simulink model "Aloe_E_Cell_Project"  (R2019b)
settings: Solver=VariableStepAuto  StartTime=0.0  StopTime=0.14  RelTol=1e-3
undefined symbols (not defined in the file): D1, Delta
libraries: powerlib x218, powerlib_meascontrol x6, simulink x2
(part 2 of 3)

== system Aloe_E_Cell_Project/Aloe E Battery Array/12 V Aloe E-Cell23 ==
  Constant : Constant  Value=4
  Constant1 : Constant  Value=24
  Controlled Current Source : powerlib/Electrical Sources/Controlled Current Source  Initialize=on  Source_Type=DC  Amplitude=1  Phase=0  Frequency=0  Measurements=None
      settings: SourceProductName=Simscape Electrical
  Controlled Voltage Source : powerlib/Electrical Sources/Controlled Voltage Source  Initialize=on  Source_Type=DC  Amplitude=1  Phase=0  Frequency=0  Measurements=Voltage
      settings: SourceProductName=Simscape Electrical
  Current Measurement : powerlib/Measurements/Current Measurement  PhasorSimulation=off  OutputType=Complex  PSBequivalent=0
      settings: SourceProductName=Simscape Electrical
  Display : Display
      settings: Decimation=3
  Display1 : Display
      settings: Decimation=3
  Series RLC Branch1 : powerlib/Elements/Series RLC Branch  LConnTagsString=__new0  RConnTagsString=__new0  BranchType=R  Resistance=6  Inductance=1e-3  SetiL0=off  InitialCurrent=0  Capacitance=1e-6  Setx0=off  InitialVoltage=0  Measurements=None
      settings: SourceProductName=Simscape Electrical
  Voltage Measurement : powerlib/Measurements/Voltage Measurement  PhasorSimulation=off  OutputType=Complex  PSBequivalent=0
      settings: SourceProductName=Simscape Electrical
  V+ : PMIOPort  Side=Right
  "V- " : PMIOPort  Port=2  Side=Right
  wires:
  Constant/1 -> Controlled Current Source/1
  Constant1/1 -> Controlled Voltage Source/1
  Current Measurement/1 -> Display1/1
  Voltage Measurement/1 -> Display/1
  connections:
  Series RLC Branch1/LConn1 -- Current Measurement/RConn1 -- Voltage Measurement/LConn1 -- V+/RConn1
  Controlled Voltage Source/RConn1 -- Controlled Current Source/LConn1
  Controlled Voltage Source/LConn1 -- Series RLC Branch1/RConn1 -- Voltage Measurement/LConn2 -- "V- "/RConn1
  Controlled Current Source/RConn1 -- Current Measurement/LConn1

== system Aloe_E_Cell_Project/Aloe E Battery Array/12 V Aloe E-Cell24 ==
  Constant : Constant  Value=4
  Constant1 : Constant  Value=24
  Controlled Current Source : powerlib/Electrical Sources/Controlled Current Source  Initialize=on  Source_Type=DC  Amplitude=1  Phase=0  Frequency=0  Measurements=None
      settings: SourceProductName=Simscape Electrical
  Controlled Voltage Source : powerlib/Electrical Sources/Controlled Voltage Source  Initialize=on  Source_Type=DC  Amplitude=1  Phase=0  Frequency=0  Measurements=Voltage
      settings: SourceProductName=Simscape Electrical
  Current Measurement : powerlib/Measurements/Current Measurement  PhasorSimulation=off  OutputType=Complex  PSBequivalent=0
      settings: SourceProductName=Simscape Electrical
  Display : Display
      settings: Decimation=3
  Display1 : Display
      settings: Decimation=3
  Series RLC Branch1 : powerlib/Elements/Series RLC Branch  LConnTagsString=__new0  RConnTagsString=__new0  BranchType=R  Resistance=6  Inductance=1e-3  SetiL0=off  InitialCurrent=0  Capacitance=1e-6  Setx0=off  InitialVoltage=0  Measurements=None
      settings: SourceProductName=Simscape Electrical
  Voltage Measurement : powerlib/Measurements/Voltage Measurement  PhasorSimulation=off  OutputType=Complex  PSBequivalent=0
      settings: SourceProductName=Simscape Electrical
  V+ : PMIOPort  Side=Right
  "V- " : PMIOPort  Port=2  Side=Right
  wires:
  Voltage Measurement/1 -> Display/1
  Current Measurement/1 -> Display1/1
  Constant1/1 -> Controlled Voltage Source/1
  Constant/1 -> Controlled Current Source/1
  connections:
  Controlled Current Source/RConn1 -- Current Measurement/LConn1
  "V- "/RConn1 -- Voltage Measurement/LConn2 -- Series RLC Branch1/RConn1 -- Controlled Voltage Source/LConn1
  Controlled Voltage Source/RConn1 -- Controlled Current Source/LConn1
  V+/RConn1 -- Voltage Measurement/LConn1 -- Current Measurement/RConn1 -- Series RLC Branch1/LConn1

== system Aloe_E_Cell_Project/Aloe E Battery Array/12 V Aloe E-Cell25 ==
  Constant : Constant  Value=4
  Constant1 : Constant  Value=24
  Controlled Current Source : powerlib/Electrical Sources/Controlled Current Source  Initialize=on  Source_Type=DC  Amplitude=1  Phase=0  Frequency=0  Measurements=None
      settings: SourceProductName=Simscape Electrical
  Controlled Voltage Source : powerlib/Electrical Sources/Controlled Voltage Source  Initialize=on  Source_Type=DC  Amplitude=1  Phase=0  Frequency=0  Measurements=Voltage
      settings: SourceProductName=Simscape Electrical
  Current Measurement : powerlib/Measurements/Current Measurement  PhasorSimulation=off  OutputType=Complex  PSBequivalent=0
      settings: SourceProductName=Simscape Electrical
  Display : Display
      settings: Decimation=3
  Display1 : Display
      settings: Decimation=3
  Series RLC Branch1 : powerlib/Elements/Series RLC Branch  LConnTagsString=__new0  RConnTagsString=__new0  BranchType=R  Resistance=6  Inductance=1e-3  SetiL0=off  InitialCurrent=0  Capacitance=1e-6  Setx0=off  InitialVoltage=0  Measurements=None
      settings: SourceProductName=Simscape Electrical
  Voltage Measurement : powerlib/Measurements/Voltage Measurement  PhasorSimulation=off  OutputType=Complex  PSBequivalent=0
      settings: SourceProductName=Simscape Electrical
  V+ : PMIOPort  Side=Right
  "V- " : PMIOPort  Port=2  Side=Right
  wires:
  Voltage Measurement/1 -> Display/1
  Current Measurement/1 -> Display1/1
  Constant1/1 -> Controlled Voltage Source/1
  Constant/1 -> Controlled Current Source/1
  connections:
  Controlled Current Source/RConn1 -- Current Measurement/LConn1
  "V- "/RConn1 -- Voltage Measurement/LConn2 -- Series RLC Branch1/RConn1 -- Controlled Voltage Source/LConn1
  Controlled Voltage Source/RConn1 -- Controlled Current Source/LConn1
  V+/RConn1 -- Voltage Measurement/LConn1 -- Current Measurement/RConn1 -- Series RLC Branch1/LConn1

== system Aloe_E_Cell_Project/Aloe E Battery Array/12 V Aloe E-Cell26 ==
  Constant : Constant  Value=4
  Constant1 : Constant  Value=24
  Controlled Current Source : powerlib/Electrical Sources/Controlled Current Source  Initialize=on  Source_Type=DC  Amplitude=1  Phase=0  Frequency=0  Measurements=None
      settings: SourceProductName=Simscape Electrical
  Controlled Voltage Source : powerlib/Electrical Sources/Controlled Voltage Source  Initialize=on  Source_Type=DC  Amplitude=1  Phase=0  Frequency=0  Measurements=Voltage
      settings: SourceProductName=Simscape Electrical
  Current Measurement : powerlib/Measurements/Current Measurement  PhasorSimulation=off  OutputType=Complex  PSBequivalent=0
      settings: SourceProductName=Simscape Electrical
  Display : Display
      settings: Decimation=3
  Display1 : Display
      settings: Decimation=3
  Series RLC Branch1 : powerlib/Elements/Series RLC Branch  LConnTagsString=__new0  RConnTagsString=__new0  BranchType=R  Resistance=6  Inductance=1e-3  SetiL0=off  InitialCurrent=0  Capacitance=1e-6  Setx0=off  InitialVoltage=0  Measurements=None
      settings: SourceProductName=Simscape Electrical
  Voltage Measurement : powerlib/Measurements/Voltage Measurement  PhasorSimulation=off  OutputType=Complex  PSBequivalent=0
      settings: SourceProductName=Simscape Electrical
  V+ : PMIOPort  Side=Right
  "V- " : PMIOPort  Port=2  Side=Right
  wires:
  Constant/1 -> Controlled Current Source/1
  Constant1/1 -> Controlled Voltage Source/1
  Current Measurement/1 -> Display1/1
  Voltage Measurement/1 -> Display/1
  connections:
  Series RLC Branch1/LConn1 -- Current Measurement/RConn1 -- Voltage Measurement/LConn1 -- V+/RConn1
  Controlled Voltage Source/RConn1 -- Controlled Current Source/LConn1
  Controlled Voltage Source/LConn1 -- Series RLC Branch1/RConn1 -- Voltage Measurement/LConn2 -- "V- "/RConn1
  Controlled Current Source/RConn1 -- Current Measurement/LConn1

== system Aloe_E_Cell_Project/Aloe E Battery Array/12 V Aloe E-Cell27 ==
  Constant : Constant  Value=4
  Constant1 : Constant  Value=24
  Controlled Current Source : powerlib/Electrical Sources/Controlled Current Source  Initialize=on  Source_Type=DC  Amplitude=1  Phase=0  Frequency=0  Measurements=None
      settings: SourceProductName=Simscape Electrical
  Controlled Voltage Source : powerlib/Electrical Sources/Controlled Voltage Source  Initialize=on  Source_Type=DC  Amplitude=1  Phase=0  Frequency=0  Measurements=Voltage
      settings: SourceProductName=Simscape Electrical
  Current Measurement : powerlib/Measurements/Current Measurement  PhasorSimulation=off  OutputType=Complex  PSBequivalent=0
      settings: SourceProductName=Simscape Electrical
  Display : Display
      settings: Decimation=3
  Display1 : Display
      settings: Decimation=3
  Series RLC Branch1 : powerlib/Elements/Series RLC Branch  LConnTagsString=__new0  RConnTagsString=__new0  BranchType=R  Resistance=6  Inductance=1e-3  SetiL0=off  InitialCurrent=0  Capacitance=1e-6  Setx0=off  InitialVoltage=0  Measurements=None
      settings: SourceProductName=Simscape Electrical
  Voltage Measurement : powerlib/Measurements/Voltage Measurement  PhasorSimulation=off  OutputType=Complex  PSBequivalent=0
      settings: SourceProductName=Simscape Electrical
  V+ : PMIOPort  Side=Right
  "V- " : PMIOPort  Port=2  Side=Right
  wires:
  Voltage Measurement/1 -> Display/1
  Current Measurement/1 -> Display1/1
  Constant1/1 -> Controlled Voltage Source/1
  Constant/1 -> Controlled Current Source/1
  connections:
  Controlled Current Source/RConn1 -- Current Measurement/LConn1
  "V- "/RConn1 -- Voltage Measurement/LConn2 -- Series RLC Branch1/RConn1 -- Controlled Voltage Source/LConn1
  Controlled Voltage Source/RConn1 -- Controlled Current Source/LConn1
  V+/RConn1 -- Voltage Measurement/LConn1 -- Current Measurement/RConn1 -- Series RLC Branch1/LConn1

== system Aloe_E_Cell_Project/Aloe E Battery Array/12 V Aloe E-Cell28 ==
  Constant : Constant  Value=4
  Constant1 : Constant  Value=24
  Controlled Current Source : powerlib/Electrical Sources/Controlled Current Source  Initialize=on  Source_Type=DC  Amplitude=1  Phase=0  Frequency=0  Measurements=None
      settings: SourceProductName=Simscape Electrical
  Controlled Voltage Source : powerlib/Electrical Sources/Controlled Voltage Source  Initialize=on  Source_Type=DC  Amplitude=1  Phase=0  Frequency=0  Measurements=Voltage
      settings: SourceProductName=Simscape Electrical
  Current Measurement : powerlib/Measurements/Current Measurement  PhasorSimulation=off  OutputType=Complex  PSBequivalent=0
      settings: SourceProductName=Simscape Electrical
  Display : Display
      settings: Decimation=3
  Display1 : Display
      settings: Decimation=3
  Series RLC Branch1 : powerlib/Elements/Series RLC Branch  LConnTagsString=__new0  RConnTagsString=__new0  BranchType=R  Resistance=6  Inductance=1e-3  SetiL0=off  InitialCurrent=0  Capacitance=1e-6  Setx0=off  InitialVoltage=0  Measurements=None
      settings: SourceProductName=Simscape Electrical
  Voltage Measurement : powerlib/Measurements/Voltage Measurement  PhasorSimulation=off  OutputType=Complex  PSBequivalent=0
      settings: SourceProductName=Simscape Electrical
  V+ : PMIOPort  Side=Right
  "V- " : PMIOPort  Port=2  Side=Right
  wires:
  Voltage Measurement/1 -> Display/1
  Current Measurement/1 -> Display1/1
  Constant1/1 -> Controlled Voltage Source/1
  Constant/1 -> Controlled Current Source/1
  connections:
  Controlled Current Source/RConn1 -- Current Measurement/LConn1
  "V- "/RConn1 -- Voltage Measurement/LConn2 -- Series RLC Branch1/RConn1 -- Controlled Voltage Source/LConn1
  Controlled Voltage Source/RConn1 -- Controlled Current Source/LConn1
  V+/RConn1 -- Voltage Measurement/LConn1 -- Current Measurement/RConn1 -- Series RLC Branch1/LConn1

== system Aloe_E_Cell_Project/Aloe E Battery Array/12 V Aloe E-Cell29 ==
  Constant : Constant  Value=4
  Constant1 : Constant  Value=24
  Controlled Current Source : powerlib/Electrical Sources/Controlled Current Source  Initialize=on  Source_Type=DC  Amplitude=1  Phase=0  Frequency=0  Measurements=None
      settings: SourceProductName=Simscape Electrical
  Controlled Voltage Source : powerlib/Electrical Sources/Controlled Voltage Source  Initialize=on  Source_Type=DC  Amplitude=1  Phase=0  Frequency=0  Measurements=Voltage
      settings: SourceProductName=Simscape Electrical
  Current Measurement : powerlib/Measurements/Current Measurement  PhasorSimulation=off  OutputType=Complex  PSBequivalent=0
      settings: SourceProductName=Simscape Electrical
  Display : Display
      settings: Decimation=3
  Display1 : Display
      settings: Decimation=3
  Series RLC Branch1 : powerlib/Elements/Series RLC Branch  LConnTagsString=__new0  RConnTagsString=__new0  BranchType=R  Resistance=6  Inductance=1e-3  SetiL0=off  InitialCurrent=0  Capacitance=1e-6  Setx0=off  InitialVoltage=0  Measurements=None
      settings: SourceProductName=Simscape Electrical
  Voltage Measurement : powerlib/Measurements/Voltage Measurement  PhasorSimulation=off  OutputType=Complex  PSBequivalent=0
      settings: SourceProductName=Simscape Electrical
  V+ : PMIOPort  Side=Right
  "V- " : PMIOPort  Port=2  Side=Right
  wires:
  Constant/1 -> Controlled Current Source/1
  Constant1/1 -> Controlled Voltage Source/1
  Current Measurement/1 -> Display1/1
  Voltage Measurement/1 -> Display/1
  connections:
  Series RLC Branch1/LConn1 -- Current Measurement/RConn1 -- Voltage Measurement/LConn1 -- V+/RConn1
  Controlled Voltage Source/RConn1 -- Controlled Current Source/LConn1
  Controlled Voltage Source/LConn1 -- Series RLC Branch1/RConn1 -- Voltage Measurement/LConn2 -- "V- "/RConn1
  Controlled Current Source/RConn1 -- Current Measurement/LConn1

== system Aloe_E_Cell_Project/Aloe E Battery Array/12 V Aloe E-Cell3 ==
  Constant : Constant  Value=4
  Constant1 : Constant  Value=24
  Controlled Current Source : powerlib/Electrical Sources/Controlled Current Source  Initialize=on  Source_Type=DC  Amplitude=1  Phase=0  Frequency=0  Measurements=None
      settings: SourceProductName=Simscape Electrical
  Controlled Voltage Source : powerlib/Electrical Sources/Controlled Voltage Source  Initialize=on  Source_Type=DC  Amplitude=1  Phase=0  Frequency=0  Measurements=Voltage
      settings: SourceProductName=Simscape Electrical
  Current Measurement : powerlib/Measurements/Current Measurement  PhasorSimulation=off  OutputType=Complex  PSBequivalent=0
      settings: SourceProductName=Simscape Electrical
  Display : Display
      settings: Decimation=3
  Display1 : Display
      settings: Decimation=3
  Series RLC Branch1 : powerlib/Elements/Series RLC Branch  LConnTagsString=__new0  RConnTagsString=__new0  BranchType=R  Resistance=6  Inductance=1e-3  SetiL0=off  InitialCurrent=0  Capacitance=1e-6  Setx0=off  InitialVoltage=0  Measurements=None
      settings: SourceProductName=Simscape Electrical
  Voltage Measurement : powerlib/Measurements/Voltage Measurement  PhasorSimulation=off  OutputType=Complex  PSBequivalent=0
      settings: SourceProductName=Simscape Electrical
  V+ : PMIOPort  Side=Right
  "V- " : PMIOPort  Port=2  Side=Right
  wires:
  Constant/1 -> Controlled Current Source/1
  Constant1/1 -> Controlled Voltage Source/1
  Current Measurement/1 -> Display1/1
  Voltage Measurement/1 -> Display/1
  connections:
  Series RLC Branch1/LConn1 -- Current Measurement/RConn1 -- Voltage Measurement/LConn1 -- V+/RConn1
  Controlled Voltage Source/RConn1 -- Controlled Current Source/LConn1
  Controlled Voltage Source/LConn1 -- Series RLC Branch1/RConn1 -- Voltage Measurement/LConn2 -- "V- "/RConn1
  Controlled Current Source/RConn1 -- Current Measurement/LConn1

== system Aloe_E_Cell_Project/Aloe E Battery Array/12 V Aloe E-Cell30 ==
  Constant : Constant  Value=4
  Constant1 : Constant  Value=24
  Controlled Current Source : powerlib/Electrical Sources/Controlled Current Source  Initialize=on  Source_Type=DC  Amplitude=1  Phase=0  Frequency=0  Measurements=None
      settings: SourceProductName=Simscape Electrical
  Controlled Voltage Source : powerlib/Electrical Sources/Controlled Voltage Source  Initialize=on  Source_Type=DC  Amplitude=1  Phase=0  Frequency=0  Measurements=Voltage
      settings: SourceProductName=Simscape Electrical
  Current Measurement : powerlib/Measurements/Current Measurement  PhasorSimulation=off  OutputType=Complex  PSBequivalent=0
      settings: SourceProductName=Simscape Electrical
  Display : Display
      settings: Decimation=3
  Display1 : Display
      settings: Decimation=3
  Series RLC Branch1 : powerlib/Elements/Series RLC Branch  LConnTagsString=__new0  RConnTagsString=__new0  BranchType=R  Resistance=6  Inductance=1e-3  SetiL0=off  InitialCurrent=0  Capacitance=1e-6  Setx0=off  InitialVoltage=0  Measurements=None
      settings: SourceProductName=Simscape Electrical
  Voltage Measurement : powerlib/Measurements/Voltage Measurement  PhasorSimulation=off  OutputType=Complex  PSBequivalent=0
      settings: SourceProductName=Simscape Electrical
  V+ : PMIOPort  Side=Right
  "V- " : PMIOPort  Port=2  Side=Right
  wires:
  Constant/1 -> Controlled Current Source/1
  Constant1/1 -> Controlled Voltage Source/1
  Current Measurement/1 -> Display1/1
  Voltage Measurement/1 -> Display/1
  connections:
  Series RLC Branch1/LConn1 -- Current Measurement/RConn1 -- Voltage Measurement/LConn1 -- V+/RConn1
  Controlled Voltage Source/RConn1 -- Controlled Current Source/LConn1
  Controlled Voltage Source/LConn1 -- Series RLC Branch1/RConn1 -- Voltage Measurement/LConn2 -- "V- "/RConn1
  Controlled Current Source/RConn1 -- Current Measurement/LConn1

== system Aloe_E_Cell_Project/Aloe E Battery Array/12 V Aloe E-Cell31 ==
  Constant : Constant  Value=4
  Constant1 : Constant  Value=24
  Controlled Current Source : powerlib/Electrical Sources/Controlled Current Source  Initialize=on  Source_Type=DC  Amplitude=1  Phase=0  Frequency=0  Measurements=None
      settings: SourceProductName=Simscape Electrical
  Controlled Voltage Source : powerlib/Electrical Sources/Controlled Voltage Source  Initialize=on  Source_Type=DC  Amplitude=1  Phase=0  Frequency=0  Measurements=Voltage
      settings: SourceProductName=Simscape Electrical
  Current Measurement : powerlib/Measurements/Current Measurement  PhasorSimulation=off  OutputType=Complex  PSBequivalent=0
      settings: SourceProductName=Simscape Electrical
  Display : Display
      settings: Decimation=3
  Display1 : Display
      settings: Decimation=3
  Series RLC Branch1 : powerlib/Elements/Series RLC Branch  LConnTagsString=__new0  RConnTagsString=__new0  BranchType=R  Resistance=6  Inductance=1e-3  SetiL0=off  InitialCurrent=0  Capacitance=1e-6  Setx0=off  InitialVoltage=0  Measurements=None
      settings: SourceProductName=Simscape Electrical
  Voltage Measurement : powerlib/Measurements/Voltage Measurement  PhasorSimulation=off  OutputType=Complex  PSBequivalent=0
      settings: SourceProductName=Simscape Electrical
  V+ : PMIOPort  Side=Right
  "V- " : PMIOPort  Port=2  Side=Right
  wires:
  Voltage Measurement/1 -> Display/1
  Current Measurement/1 -> Display1/1
  Constant1/1 -> Controlled Voltage Source/1
  Constant/1 -> Controlled Current Source/1
  connections:
  Controlled Current Source/RConn1 -- Current Measurement/LConn1
  "V- "/RConn1 -- Voltage Measurement/LConn2 -- Series RLC Branch1/RConn1 -- Controlled Voltage Source/LConn1
  Controlled Voltage Source/RConn1 -- Controlled Current Source/LConn1
  V+/RConn1 -- Voltage Measurement/LConn1 -- Current Measurement/RConn1 -- Series RLC Branch1/LConn1

== system Aloe_E_Cell_Project/Aloe E Battery Array/12 V Aloe E-Cell32 ==
  Constant : Constant  Value=4
  Constant1 : Constant  Value=24
  Controlled Current Source : powerlib/Electrical Sources/Controlled Current Source  Initialize=on  Source_Type=DC  Amplitude=1  Phase=0  Frequency=0  Measurements=None
      settings: SourceProductName=Simscape Electrical
  Controlled Voltage Source : powerlib/Electrical Sources/Controlled Voltage Source  Initialize=on  Source_Type=DC  Amplitude=1  Phase=0  Frequency=0  Measurements=Voltage
      settings: SourceProductName=Simscape Electrical
  Current Measurement : powerlib/Measurements/Current Measurement  PhasorSimulation=off  OutputType=Complex  PSBequivalent=0
      settings: SourceProductName=Simscape Electrical
  Display : Display
      settings: Decimation=3
  Display1 : Display
      settings: Decimation=3
  Series RLC Branch1 : powerlib/Elements/Series RLC Branch  LConnTagsString=__new0  RConnTagsString=__new0  BranchType=R  Resistance=6  Inductance=1e-3  SetiL0=off  InitialCurrent=0  Capacitance=1e-6  Setx0=off  InitialVoltage=0  Measurements=None
      settings: SourceProductName=Simscape Electrical
  Voltage Measurement : powerlib/Measurements/Voltage Measurement  PhasorSimulation=off  OutputType=Complex  PSBequivalent=0
      settings: SourceProductName=Simscape Electrical
  V+ : PMIOPort  Side=Right
  "V- " : PMIOPort  Port=2  Side=Right
  wires:
  Constant/1 -> Controlled Current Source/1
  Constant1/1 -> Controlled Voltage Source/1
  Current Measurement/1 -> Display1/1
  Voltage Measurement/1 -> Display/1
  connections:
  Series RLC Branch1/LConn1 -- Current Measurement/RConn1 -- Voltage Measurement/LConn1 -- V+/RConn1
  Controlled Voltage Source/RConn1 -- Controlled Current Source/LConn1
  Controlled Voltage Source/LConn1 -- Series RLC Branch1/RConn1 -- Voltage Measurement/LConn2 -- "V- "/RConn1
  Controlled Current Source/RConn1 -- Current Measurement/LConn1

== system Aloe_E_Cell_Project/Aloe E Battery Array/12 V Aloe E-Cell33 ==
  Constant : Constant  Value=4
  Constant1 : Constant  Value=24
  Controlled Current Source : powerlib/Electrical Sources/Controlled Current Source  Initialize=on  Source_Type=DC  Amplitude=1  Phase=0  Frequency=0  Measurements=None
      settings: SourceProductName=Simscape Electrical
  Controlled Voltage Source : powerlib/Electrical Sources/Controlled Voltage Source  Initialize=on  Source_Type=DC  Amplitude=1  Phase=0  Frequency=0  Measurements=Voltage
      settings: SourceProductName=Simscape Electrical
  Current Measurement : powerlib/Measurements/Current Measurement  PhasorSimulation=off  OutputType=Complex  PSBequivalent=0
      settings: SourceProductName=Simscape Electrical
  Display : Display
      settings: Decimation=3
  Display1 : Display
      settings: Decimation=3
  Series RLC Branch1 : powerlib/Elements/Series RLC Branch  LConnTagsString=__new0  RConnTagsString=__new0  BranchType=R  Resistance=6  Inductance=1e-3  SetiL0=off  InitialCurrent=0  Capacitance=1e-6  Setx0=off  InitialVoltage=0  Measurements=None
      settings: SourceProductName=Simscape Electrical
  Voltage Measurement : powerlib/Measurements/Voltage Measurement  PhasorSimulation=off  OutputType=Complex  PSBequivalent=0
      settings: SourceProductName=Simscape Electrical
  V+ : PMIOPort  Side=Right
  "V- " : PMIOPort  Port=2  Side=Right
  wires:
  Constant/1 -> Controlled Current Source/1
  Constant1/1 -> Controlled Voltage Source/1
  Current Measurement/1 -> Display1/1
  Voltage Measurement/1 -> Display/1
  connections:
  Series RLC Branch1/LConn1 -- Current Measurement/RConn1 -- Voltage Measurement/LConn1 -- V+/RConn1
  Controlled Voltage Source/RConn1 -- Controlled Current Source/LConn1
  Controlled Voltage Source/LConn1 -- Series RLC Branch1/RConn1 -- Voltage Measurement/LConn2 -- "V- "/RConn1
  Controlled Current Source/RConn1 -- Current Measurement/LConn1

== system Aloe_E_Cell_Project/Aloe E Battery Array/12 V Aloe E-Cell34 ==
  Constant : Constant  Value=4
  Constant1 : Constant  Value=24
  Controlled Current Source : powerlib/Electrical Sources/Controlled Current Source  Initialize=on  Source_Type=DC  Amplitude=1  Phase=0  Frequency=0  Measurements=None
      settings: SourceProductName=Simscape Electrical
  Controlled Voltage Source : powerlib/Electrical Sources/Controlled Voltage Source  Initialize=on  Source_Type=DC  Amplitude=1  Phase=0  Frequency=0  Measurements=Voltage
      settings: SourceProductName=Simscape Electrical
  Current Measurement : powerlib/Measurements/Current Measurement  PhasorSimulation=off  OutputType=Complex  PSBequivalent=0
      settings: SourceProductName=Simscape Electrical
  Display : Display
      settings: Decimation=3
  Display1 : Display
      settings: Decimation=3
  Series RLC Branch1 : powerlib/Elements/Series RLC Branch  LConnTagsString=__new0  RConnTagsString=__new0  BranchType=R  Resistance=6  Inductance=1e-3  SetiL0=off  InitialCurrent=0  Capacitance=1e-6  Setx0=off  InitialVoltage=0  Measurements=None
      settings: SourceProductName=Simscape Electrical
  Voltage Measurement : powerlib/Measurements/Voltage Measurement  PhasorSimulation=off  OutputType=Complex  PSBequivalent=0
      settings: SourceProductName=Simscape Electrical
  V+ : PMIOPort  Side=Right
  "V- " : PMIOPort  Port=2  Side=Right
  wires:
  Voltage Measurement/1 -> Display/1
  Current Measurement/1 -> Display1/1
  Constant1/1 -> Controlled Voltage Source/1
  Constant/1 -> Controlled Current Source/1
  connections:
  Controlled Current Source/RConn1 -- Current Measurement/LConn1
  "V- "/RConn1 -- Voltage Measurement/LConn2 -- Series RLC Branch1/RConn1 -- Controlled Voltage Source/LConn1
  Controlled Voltage Source/RConn1 -- Controlled Current Source/LConn1
  V+/RConn1 -- Voltage Measurement/LConn1 -- Current Measurement/RConn1 -- Series RLC Branch1/LConn1

== system Aloe_E_Cell_Project/Aloe E Battery Array/12 V Aloe E-Cell35 ==
  Constant : Constant  Value=4
  Constant1 : Constant  Value=24
  Controlled Current Source : powerlib/Electrical Sources/Controlled Current Source  Initialize=on  Source_Type=DC  Amplitude=1  Phase=0  Frequency=0  Measurements=None
      settings: SourceProductName=Simscape Electrical
  Controlled Voltage Source : powerlib/Electrical Sources/Controlled Voltage Source  Initialize=on  Source_Type=DC  Amplitude=1  Phase=0  Frequency=0  Measurements=Voltage
      settings: SourceProductName=Simscape Electrical
  Current Measurement : powerlib/Measurements/Current Measurement  PhasorSimulation=off  OutputType=Complex  PSBequivalent=0
      settings: SourceProductName=Simscape Electrical
  Display : Display
      settings: Decimation=3
  Display1 : Display
      settings: Decimation=3
  Series RLC Branch1 : powerlib/Elements/Series RLC Branch  LConnTagsString=__new0  RConnTagsString=__new0  BranchType=R  Resistance=6  Inductance=1e-3  SetiL0=off  InitialCurrent=0  Capacitance=1e-6  Setx0=off  InitialVoltage=0  Measurements=None
      settings: SourceProductName=Simscape Electrical
  Voltage Measurement : powerlib/Measurements/Voltage Measurement  PhasorSimulation=off  OutputType=Complex  PSBequivalent=0
      settings: SourceProductName=Simscape Electrical
  V+ : PMIOPort  Side=Right
  "V- " : PMIOPort  Port=2  Side=Right
  wires:
  Constant/1 -> Controlled Current Source/1
  Constant1/1 -> Controlled Voltage Source/1
  Current Measurement/1 -> Display1/1
  Voltage Measurement/1 -> Display/1
  connections:
  Series RLC Branch1/LConn1 -- Current Measurement/RConn1 -- Voltage Measurement/LConn1 -- V+/RConn1
  Controlled Voltage Source/RConn1 -- Controlled Current Source/LConn1
  Controlled Voltage Source/LConn1 -- Series RLC Branch1/RConn1 -- Voltage Measurement/LConn2 -- "V- "/RConn1
  Controlled Current Source/RConn1 -- Current Measurement/LConn1

== system Aloe_E_Cell_Project/Aloe E Battery Array/12 V Aloe E-Cell36 ==
  Constant : Constant  Value=4
  Constant1 : Constant  Value=24
  Controlled Current Source : powerlib/Electrical Sources/Controlled Current Source  Initialize=on  Source_Type=DC  Amplitude=1  Phase=0  Frequency=0  Measurements=None
      settings: SourceProductName=Simscape Electrical
  Controlled Voltage Source : powerlib/Electrical Sources/Controlled Voltage Source  Initialize=on  Source_Type=DC  Amplitude=1  Phase=0  Frequency=0  Measurements=Voltage
      settings: SourceProductName=Simscape Electrical
  Current Measurement : powerlib/Measurements/Current Measurement  PhasorSimulation=off  OutputType=Complex  PSBequivalent=0
      settings: SourceProductName=Simscape Electrical
  Display : Display
      settings: Decimation=3
  Display1 : Display
      settings: Decimation=3
  Series RLC Branch1 : powerlib/Elements/Series RLC Branch  LConnTagsString=__new0  RConnTagsString=__new0  BranchType=R  Resistance=6  Inductance=1e-3  SetiL0=off  InitialCurrent=0  Capacitance=1e-6  Setx0=off  InitialVoltage=0  Measurements=None
      settings: SourceProductName=Simscape Electrical
  Voltage Measurement : powerlib/Measurements/Voltage Measurement  PhasorSimulation=off  OutputType=Complex  PSBequivalent=0
      settings: SourceProductName=Simscape Electrical
  V+ : PMIOPort  Side=Right
  "V- " : PMIOPort  Port=2  Side=Right
  wires:
  Constant/1 -> Controlled Current Source/1
  Constant1/1 -> Controlled Voltage Source/1
  Current Measurement/1 -> Display1/1
  Voltage Measurement/1 -> Display/1
  connections:
  Series RLC Branch1/LConn1 -- Current Measurement/RConn1 -- Voltage Measurement/LConn1 -- V+/RConn1
  Controlled Voltage Source/RConn1 -- Controlled Current Source/LConn1
  Controlled Voltage Source/LConn1 -- Series RLC Branch1/RConn1 -- Voltage Measurement/LConn2 -- "V- "/RConn1
  Controlled Current Source/RConn1 -- Current Measurement/LConn1

== system Aloe_E_Cell_Project/Aloe E Battery Array/12 V Aloe E-Cell37 ==
  Constant : Constant  Value=4
  Constant1 : Constant  Value=24
  Controlled Current Source : powerlib/Electrical Sources/Controlled Current Source  Initialize=on  Source_Type=DC  Amplitude=1  Phase=0  Frequency=0  Measurements=None
      settings: SourceProductName=Simscape Electrical
  Controlled Voltage Source : powerlib/Electrical Sources/Controlled Voltage Source  Initialize=on  Source_Type=DC  Amplitude=1  Phase=0  Frequency=0  Measurements=Voltage
      settings: SourceProductName=Simscape Electrical
  Current Measurement : powerlib/Measurements/Current Measurement  PhasorSimulation=off  OutputType=Complex  PSBequivalent=0
      settings: SourceProductName=Simscape Electrical
  Display : Display
      settings: Decimation=3
  Display1 : Display
      settings: Decimation=3
  Series RLC Branch1 : powerlib/Elements/Series RLC Branch  LConnTagsString=__new0  RConnTagsString=__new0  BranchType=R  Resistance=6  Inductance=1e-3  SetiL0=off  InitialCurrent=0  Capacitance=1e-6  Setx0=off  InitialVoltage=0  Measurements=None
      settings: SourceProductName=Simscape Electrical
  Voltage Measurement : powerlib/Measurements/Voltage Measurement  PhasorSimulation=off  OutputType=Complex  PSBequivalent=0
      settings: SourceProductName=Simscape Electrical
  V+ : PMIOPort  Side=Right
  "V- " : PMIOPort  Port=2  Side=Right
  wires:
  Voltage Measurement/1 -> Display/1
  Current Measurement/1 -> Display1/1
  Constant1/1 -> Controlled Voltage Source/1
  Constant/1 -> Controlled Current Source/1
  connections:
  Controlled Current Source/RConn1 -- Current Measurement/LConn1
  "V- "/RConn1 -- Voltage Measurement/LConn2 -- Series RLC Branch1/RConn1 -- Controlled Voltage Source/LConn1
  Controlled Voltage Source/RConn1 -- Controlled Current Source/LConn1
  V+/RConn1 -- Voltage Measurement/LConn1 -- Current Measurement/RConn1 -- Series RLC Branch1/LConn1

== system Aloe_E_Cell_Project/Aloe E Battery Array/12 V Aloe E-Cell38 ==
  Constant : Constant  Value=4
  Constant1 : Constant  Value=24
  Controlled Current Source : powerlib/Electrical Sources/Controlled Current Source  Initialize=on  Source_Type=DC  Amplitude=1  Phase=0  Frequency=0  Measurements=None
      settings: SourceProductName=Simscape Electrical
  Controlled Voltage Source : powerlib/Electrical Sources/Controlled Voltage Source  Initialize=on  Source_Type=DC  Amplitude=1  Phase=0  Frequency=0  Measurements=Voltage
      settings: SourceProductName=Simscape Electrical
  Current Measurement : powerlib/Measurements/Current Measurement  PhasorSimulation=off  OutputType=Complex  PSBequivalent=0
      settings: SourceProductName=Simscape Electrical
  Display : Display
      settings: Decimation=3
  Display1 : Display
      settings: Decimation=3
  Series RLC Branch1 : powerlib/Elements/Series RLC Branch  LConnTagsString=__new0  RConnTagsString=__new0  BranchType=R  Resistance=6  Inductance=1e-3  SetiL0=off  InitialCurrent=0  Capacitance=1e-6  Setx0=off  InitialVoltage=0  Measurements=None
      settings: SourceProductName=Simscape Electrical
  Voltage Measurement : powerlib/Measurements/Voltage Measurement  PhasorSimulation=off  OutputType=Complex  PSBequivalent=0
      settings: SourceProductName=Simscape Electrical
  V+ : PMIOPort  Side=Right
  "V- " : PMIOPort  Port=2  Side=Right
  wires:
  Voltage Measurement/1 -> Display/1
  Current Measurement/1 -> Display1/1
  Constant1/1 -> Controlled Voltage Source/1
  Constant/1 -> Controlled Current Source/1
  connections:
  Controlled Current Source/RConn1 -- Current Measurement/LConn1
  "V- "/RConn1 -- Voltage Measurement/LConn2 -- Series RLC Branch1/RConn1 -- Controlled Voltage Source/LConn1
  Controlled Voltage Source/RConn1 -- Controlled Current Source/LConn1
  V+/RConn1 -- Voltage Measurement/LConn1 -- Current Measurement/RConn1 -- Series RLC Branch1/LConn1

== system Aloe_E_Cell_Project/Aloe E Battery Array/12 V Aloe E-Cell39 ==
  Constant : Constant  Value=4
  Constant1 : Constant  Value=24
  Controlled Current Source : powerlib/Electrical Sources/Controlled Current Source  Initialize=on  Source_Type=DC  Amplitude=1  Phase=0  Frequency=0  Measurements=None
      settings: SourceProductName=Simscape Electrical
  Controlled Voltage Source : powerlib/Electrical Sources/Controlled Voltage Source  Initialize=on  Source_Type=DC  Amplitude=1  Phase=0  Frequency=0  Measurements=Voltage
      settings: SourceProductName=Simscape Electrical
  Current Measurement : powerlib/Measurements/Current Measurement  PhasorSimulation=off  OutputType=Complex  PSBequivalent=0
      settings: SourceProductName=Simscape Electrical
  Display : Display
      settings: Decimation=3
  Display1 : Display
      settings: Decimation=3
  Series RLC Branch1 : powerlib/Elements/Series RLC Branch  LConnTagsString=__new0  RConnTagsString=__new0  BranchType=R  Resistance=6  Inductance=1e-3  SetiL0=off  InitialCurrent=0  Capacitance=1e-6  Setx0=off  InitialVoltage=0  Measurements=None
      settings: SourceProductName=Simscape Electrical
  Voltage Measurement : powerlib/Measurements/Voltage Measurement  PhasorSimulation=off  OutputType=Complex  PSBequivalent=0
      settings: SourceProductName=Simscape Electrical
  V+ : PMIOPort  Side=Right
  "V- " : PMIOPort  Port=2  Side=Right
  wires:
  Constant/1 -> Controlled Current Source/1
  Constant1/1 -> Controlled Voltage Source/1
  Current Measurement/1 -> Display1/1
  Voltage Measurement/1 -> Display/1
  connections:
  Series RLC Branch1/LConn1 -- Current Measurement/RConn1 -- Voltage Measurement/LConn1 -- V+/RConn1
  Controlled Voltage Source/RConn1 -- Controlled Current Source/LConn1
  Controlled Voltage Source/LConn1 -- Series RLC Branch1/RConn1 -- Voltage Measurement/LConn2 -- "V- "/RConn1
  Controlled Current Source/RConn1 -- Current Measurement/LConn1

== system Aloe_E_Cell_Project/Aloe E Battery Array/12 V Aloe E-Cell4 ==
  Constant : Constant  Value=4
  Constant1 : Constant  Value=24
  Controlled Current Source : powerlib/Electrical Sources/Controlled Current Source  Initialize=on  Source_Type=DC  Amplitude=1  Phase=0  Frequency=0  Measurements=None
      settings: SourceProductName=Simscape Electrical
  Controlled Voltage Source : powerlib/Electrical Sources/Controlled Voltage Source  Initialize=on  Source_Type=DC  Amplitude=1  Phase=0  Frequency=0  Measurements=Voltage
      settings: SourceProductName=Simscape Electrical
  Current Measurement : powerlib/Measurements/Current Measurement  PhasorSimulation=off  OutputType=Complex  PSBequivalent=0
      settings: SourceProductName=Simscape Electrical
  Display : Display
      settings: Decimation=3
  Display1 : Display
      settings: Decimation=3
  Series RLC Branch1 : powerlib/Elements/Series RLC Branch  LConnTagsString=__new0  RConnTagsString=__new0  BranchType=R  Resistance=6  Inductance=1e-3  SetiL0=off  InitialCurrent=0  Capacitance=1e-6  Setx0=off  InitialVoltage=0  Measurements=None
      settings: SourceProductName=Simscape Electrical
  Voltage Measurement : powerlib/Measurements/Voltage Measurement  PhasorSimulation=off  OutputType=Complex  PSBequivalent=0
      settings: SourceProductName=Simscape Electrical
  V+ : PMIOPort  Side=Right
  "V- " : PMIOPort  Port=2  Side=Right
  wires:
  Voltage Measurement/1 -> Display/1
  Current Measurement/1 -> Display1/1
  Constant1/1 -> Controlled Voltage Source/1
  Constant/1 -> Controlled Current Source/1
  connections:
  Controlled Current Source/RConn1 -- Current Measurement/LConn1
  "V- "/RConn1 -- Voltage Measurement/LConn2 -- Series RLC Branch1/RConn1 -- Controlled Voltage Source/LConn1
  Controlled Voltage Source/RConn1 -- Controlled Current Source/LConn1
  V+/RConn1 -- Voltage Measurement/LConn1 -- Current Measurement/RConn1 -- Series RLC Branch1/LConn1

== system Aloe_E_Cell_Project/Aloe E Battery Array/12 V Aloe E-Cell40 ==
  Constant : Constant  Value=4
  Constant1 : Constant  Value=24
  Controlled Current Source : powerlib/Electrical Sources/Controlled Current Source  Initialize=on  Source_Type=DC  Amplitude=1  Phase=0  Frequency=0  Measurements=None
      settings: SourceProductName=Simscape Electrical
  Controlled Voltage Source : powerlib/Electrical Sources/Controlled Voltage Source  Initialize=on  Source_Type=DC  Amplitude=1  Phase=0  Frequency=0  Measurements=Voltage
      settings: SourceProductName=Simscape Electrical
  Current Measurement : powerlib/Measurements/Current Measurement  PhasorSimulation=off  OutputType=Complex  PSBequivalent=0
      settings: SourceProductName=Simscape Electrical
  Display : Display
      settings: Decimation=3
  Display1 : Display
      settings: Decimation=3
  Series RLC Branch1 : powerlib/Elements/Series RLC Branch  LConnTagsString=__new0  RConnTagsString=__new0  BranchType=R  Resistance=6  Inductance=1e-3  SetiL0=off  InitialCurrent=0  Capacitance=1e-6  Setx0=off  InitialVoltage=0  Measurements=None
      settings: SourceProductName=Simscape Electrical
  Voltage Measurement : powerlib/Measurements/Voltage Measurement  PhasorSimulation=off  OutputType=Complex  PSBequivalent=0
      settings: SourceProductName=Simscape Electrical
  V+ : PMIOPort  Side=Right
  "V- " : PMIOPort  Port=2  Side=Right
  wires:
  Voltage Measurement/1 -> Display/1
  Current Measurement/1 -> Display1/1
  Constant1/1 -> Controlled Voltage Source/1
  Constant/1 -> Controlled Current Source/1
  connections:
  Controlled Current Source/RConn1 -- Current Measurement/LConn1
  "V- "/RConn1 -- Voltage Measurement/LConn2 -- Series RLC Branch1/RConn1 -- Controlled Voltage Source/LConn1
  Controlled Voltage Source/RConn1 -- Controlled Current Source/LConn1
  V+/RConn1 -- Voltage Measurement/LConn1 -- Current Measurement/RConn1 -- Series RLC Branch1/LConn1

== system Aloe_E_Cell_Project/Aloe E Battery Array/12 V Aloe E-Cell5 ==
  Constant : Constant  Value=4
  Constant1 : Constant  Value=24
  Controlled Current Source : powerlib/Electrical Sources/Controlled Current Source  Initialize=on  Source_Type=DC  Amplitude=1  Phase=0  Frequency=0  Measurements=None
      settings: SourceProductName=Simscape Electrical
  Controlled Voltage Source : powerlib/Electrical Sources/Controlled Voltage Source  Initialize=on  Source_Type=DC  Amplitude=1  Phase=0  Frequency=0  Measurements=Voltage
      settings: SourceProductName=Simscape Electrical
  Current Measurement : powerlib/Measurements/Current Measurement  PhasorSimulation=off  OutputType=Complex  PSBequivalent=0
      settings: SourceProductName=Simscape Electrical
  Display : Display
      settings: Decimation=3
  Display1 : Display
      settings: Decimation=3
  Series RLC Branch1 : powerlib/Elements/Series RLC Branch  LConnTagsString=__new0  RConnTagsString=__new0  BranchType=R  Resistance=6  Inductance=1e-3  SetiL0=off  InitialCurrent=0  Capacitance=1e-6  Setx0=off  InitialVoltage=0  Measurements=None
      settings: SourceProductName=Simscape Electrical
  Voltage Measurement : powerlib/Measurements/Voltage Measurement  PhasorSimulation=off  OutputType=Complex  PSBequivalent=0
      settings: SourceProductName=Simscape Electrical
  V+ : PMIOPort  Side=Right
  "V- " : PMIOPort  Port=2  Side=Right
  wires:
  Voltage Measurement/1 -> Display/1
  Current Measurement/1 -> Display1/1
  Constant1/1 -> Controlled Voltage Source/1
  Constant/1 -> Controlled Current Source/1
  connections:
  Controlled Current Source/RConn1 -- Current Measurement/LConn1
  "V- "/RConn1 -- Voltage Measurement/LConn2 -- Series RLC Branch1/RConn1 -- Controlled Voltage Source/LConn1
  Controlled Voltage Source/RConn1 -- Controlled Current Source/LConn1
  V+/RConn1 -- Voltage Measurement/LConn1 -- Current Measurement/RConn1 -- Series RLC Branch1/LConn1

== system Aloe_E_Cell_Project/Aloe E Battery Array/12 V Aloe E-Cell6 ==
  Constant : Constant  Value=4
  Constant1 : Constant  Value=24
  Controlled Current Source : powerlib/Electrical Sources/Controlled Current Source  Initialize=on  Source_Type=DC  Amplitude=1  Phase=0  Frequency=0  Measurements=None
      settings: SourceProductName=Simscape Electrical
  Controlled Voltage Source : powerlib/Electrical Sources/Controlled Voltage Source  Initialize=on  Source_Type=DC  Amplitude=1  Phase=0  Frequency=0  Measurements=Voltage
      settings: SourceProductName=Simscape Electrical
  Current Measurement : powerlib/Measurements/Current Measurement  PhasorSimulation=off  OutputType=Complex  PSBequivalent=0
      settings: SourceProductName=Simscape Electrical
  Display : Display
      settings: Decimation=3
  Display1 : Display
      settings: Decimation=3
  Series RLC Branch1 : powerlib/Elements/Series RLC Branch  LConnTagsString=__new0  RConnTagsString=__new0  BranchType=R  Resistance=6  Inductance=1e-3  SetiL0=off  InitialCurrent=0  Capacitance=1e-6  Setx0=off  InitialVoltage=0  Measurements=None
      settings: SourceProductName=Simscape Electrical
  Voltage Measurement : powerlib/Measurements/Voltage Measurement  PhasorSimulation=off  OutputType=Complex  PSBequivalent=0
      settings: SourceProductName=Simscape Electrical
  V+ : PMIOPort  Side=Right
  "V- " : PMIOPort  Port=2  Side=Right
  wires:
  Constant/1 -> Controlled Current Source/1
  Constant1/1 -> Controlled Voltage Source/1
  Current Measurement/1 -> Display1/1
  Voltage Measurement/1 -> Display/1
  connections:
  Series RLC Branch1/LConn1 -- Current Measurement/RConn1 -- Voltage Measurement/LConn1 -- V+/RConn1
  Controlled Voltage Source/RConn1 -- Controlled Current Source/LConn1
  Controlled Voltage Source/LConn1 -- Series RLC Branch1/RConn1 -- Voltage Measurement/LConn2 -- "V- "/RConn1
  Controlled Current Source/RConn1 -- Current Measurement/LConn1

== system Aloe_E_Cell_Project/Aloe E Battery Array/12 V Aloe E-Cell7 ==
  Constant : Constant  Value=4
  Constant1 : Constant  Value=24
  Controlled Current Source : powerlib/Electrical Sources/Controlled Current Source  Initialize=on  Source_Type=DC  Amplitude=1  Phase=0  Frequency=0  Measurements=None
      settings: SourceProductName=Simscape Electrical
  Controlled Voltage Source : powerlib/Electrical Sources/Controlled Voltage Source  Initialize=on  Source_Type=DC  Amplitude=1  Phase=0  Frequency=0  Measurements=Voltage
      settings: SourceProductName=Simscape Electrical
  Current Measurement : powerlib/Measurements/Current Measurement  PhasorSimulation=off  OutputType=Complex  PSBequivalent=0
      settings: SourceProductName=Simscape Electrical
  Display : Display
      settings: Decimation=3
  Display1 : Display
      settings: Decimation=3
  Series RLC Branch1 : powerlib/Elements/Series RLC Branch  LConnTagsString=__new0  RConnTagsString=__new0  BranchType=R  Resistance=6  Inductance=1e-3  SetiL0=off  InitialCurrent=0  Capacitance=1e-6  Setx0=off  InitialVoltage=0  Measurements=None
      settings: SourceProductName=Simscape Electrical
  Voltage Measurement : powerlib/Measurements/Voltage Measurement  PhasorSimulation=off  OutputType=Complex  PSBequivalent=0
      settings: SourceProductName=Simscape Electrical
  V+ : PMIOPort  Side=Right
  "V- " : PMIOPort  Port=2  Side=Right
  wires:
  Constant/1 -> Controlled Current Source/1
  Constant1/1 -> Controlled Voltage Source/1
  Current Measurement/1 -> Display1/1
  Voltage Measurement/1 -> Display/1
  connections:
  Series RLC Branch1/LConn1 -- Current Measurement/RConn1 -- Voltage Measurement/LConn1 -- V+/RConn1
  Controlled Voltage Source/RConn1 -- Controlled Current Source/LConn1
  Controlled Voltage Source/LConn1 -- Series RLC Branch1/RConn1 -- Voltage Measurement/LConn2 -- "V- "/RConn1
  Controlled Current Source/RConn1 -- Current Measurement/LConn1

== system Aloe_E_Cell_Project/Aloe E Battery Array/12 V Aloe E-Cell8 ==
  Constant : Constant  Value=4
  Constant1 : Constant  Value=24
  Controlled Current Source : powerlib/Electrical Sources/Controlled Current Source  Initialize=on  Source_Type=DC  Amplitude=1  Phase=0  Frequency=0  Measurements=None
      settings: SourceProductName=Simscape Electrical
  Controlled Voltage Source : powerlib/Electrical Sources/Controlled Voltage Source  Initialize=on  Source_Type=DC  Amplitude=1  Phase=0  Frequency=0  Measurements=Voltage
      settings: SourceProductName=Simscape Electrical
  Current Measurement : powerlib/Measurements/Current Measurement  PhasorSimulation=off  OutputType=Complex  PSBequivalent=0
      settings: SourceProductName=Simscape Electrical
  Display : Display
      settings: Decimation=3
  Display1 : Display
      settings: Decimation=3
  Series RLC Branch1 : powerlib/Elements/Series RLC Branch  LConnTagsString=__new0  RConnTagsString=__new0  BranchType=R  Resistance=6  Inductance=1e-3  SetiL0=off  InitialCurrent=0  Capacitance=1e-6  Setx0=off  InitialVoltage=0  Measurements=None
      settings: SourceProductName=Simscape Electrical
  Voltage Measurement : powerlib/Measurements/Voltage Measurement  PhasorSimulation=off  OutputType=Complex  PSBequivalent=0
      settings: SourceProductName=Simscape Electrical
  V+ : PMIOPort  Side=Right
  "V- " : PMIOPort  Port=2  Side=Right
  wires:
  Voltage Measurement/1 -> Display/1
  Current Measurement/1 -> Display1/1
  Constant1/1 -> Controlled Voltage Source/1
  Constant/1 -> Controlled Current Source/1
  connections:
  Controlled Current Source/RConn1 -- Current Measurement/LConn1
  "V- "/RConn1 -- Voltage Measurement/LConn2 -- Series RLC Branch1/RConn1 -- Controlled Voltage Source/LConn1
  Controlled Voltage Source/RConn1 -- Controlled Current Source/LConn1
  V+/RConn1 -- Voltage Measurement/LConn1 -- Current Measurement/RConn1 -- Series RLC Branch1/LConn1

== system Aloe_E_Cell_Project/Aloe E Battery Array/12 V Aloe E-Cell9 ==
  Constant : Constant  Value=4
  Constant1 : Constant  Value=24
  Controlled Current Source : powerlib/Electrical Sources/Controlled Current Source  Initialize=on  Source_Type=DC  Amplitude=1  Phase=0  Frequency=0  Measurements=None
      settings: SourceProductName=Simscape Electrical
  Controlled Voltage Source : powerlib/Electrical Sources/Controlled Voltage Source  Initialize=on  Source_Type=DC  Amplitude=1  Phase=0  Frequency=0  Measurements=Voltage
      settings: SourceProductName=Simscape Electrical
  Current Measurement : powerlib/Measurements/Current Measurement  PhasorSimulation=off  OutputType=Complex  PSBequivalent=0
      settings: SourceProductName=Simscape Electrical
  Display : Display
      settings: Decimation=3
  Display1 : Display
      settings: Decimation=3
  Series RLC Branch1 : powerlib/Elements/Series RLC Branch  LConnTagsString=__new0  RConnTagsString=__new0  BranchType=R  Resistance=6  Inductance=1e-3  SetiL0=off  InitialCurrent=0  Capacitance=1e-6  Setx0=off  InitialVoltage=0  Measurements=None
      settings: SourceProductName=Simscape Electrical
  Voltage Measurement : powerlib/Measurements/Voltage Measurement  PhasorSimulation=off  OutputType=Complex  PSBequivalent=0
      settings: SourceProductName=Simscape Electrical
  V+ : PMIOPort  Side=Right
  "V- " : PMIOPort  Port=2  Side=Right
  wires:
  Constant/1 -> Controlled Current Source/1
  Constant1/1 -> Controlled Voltage Source/1
  Current Measurement/1 -> Display1/1
  Voltage Measurement/1 -> Display/1
  connections:
  Series RLC Branch1/LConn1 -- Current Measurement/RConn1 -- Voltage Measurement/LConn1 -- V+/RConn1
  Controlled Voltage Source/RConn1 -- Controlled Current Source/LConn1
  Controlled Voltage Source/LConn1 -- Series RLC Branch1/RConn1 -- Voltage Measurement/LConn2 -- "V- "/RConn1
  Controlled Current Source/RConn1 -- Current Measurement/LConn1
